simulink model "threshold_single"  (Simulink 5.0)
settings: Solver=ode45  StartTime=0.0  StopTime=10.0  RelTol=1e-3
settings Model: LastModifiedBy=Administrator

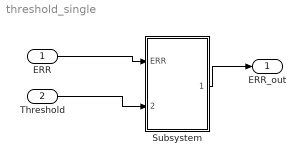
== system threshold_single ==
  ERR : Inport
  Threshold : Inport  Port=2
  Subsystem : Subsystem
  ERR_out : Outport
  wires:
  ERR/1 -> Subsystem/1(ERR)
  Subsystem/1(ERR_out) -> ERR_out/1
  Threshold/1 -> Subsystem/2(THRESHOLD)

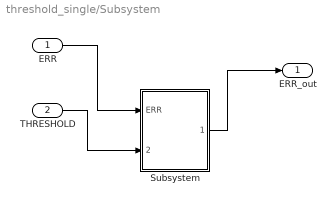
== system threshold_single/Subsystem ==
  ERR : Inport
  THRESHOLD : Inport  Port=2
  Subsystem : Subsystem  mask{T=400e-6}
      mask prompts: T "Threshold"
  ERR_out : Outport
  wires:
  ERR/1 -> Subsystem/1(ERR)
  Subsystem/1(ERR_out) -> ERR_out/1
  THRESHOLD/1 -> Subsystem/2(THRESHOLD)

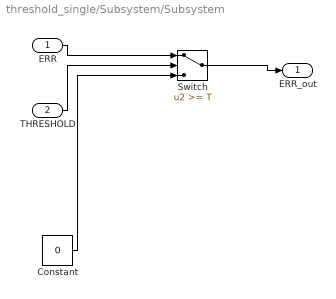
== system threshold_single/Subsystem/Subsystem ==
  ERR : Inport
  THRESHOLD : Inport  Port=2
  Constant : Constant  Value=0
  Switch : Switch  Threshold=T  SaturateOnIntegerOverflow=on
  ERR_out : Outport
  wires:
  ERR/1 -> Switch/1
  THRESHOLD/1 -> Switch/2
  Switch/1 -> ERR_out/1
  Constant/1 -> Switch/3
